simulink model "simulinkBUCK"  (R2022b)
settings: Solver=ode45  StartTime=0.0  StopTime=0.01  RelTol=1e-3
values from neighbouring files (symbols this model uses):
  C = 10e-6    (= 1e-05)    [BUCK_Parameters.m]
  L = 0.002    [BUCK_Parameters.m]
  R = 10    [BUCK_Parameters.m]
  Vin = 32    [BUCK_Parameters.m]
settings Model: Creator=ferch  LastModifiedBy=ferch

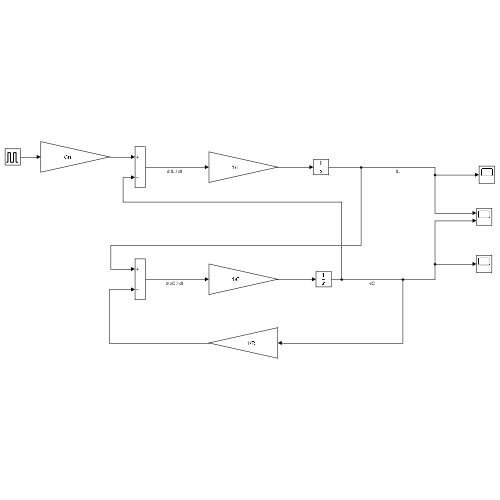
[thumbnail: Simulink's stored preview of the top-level diagram]
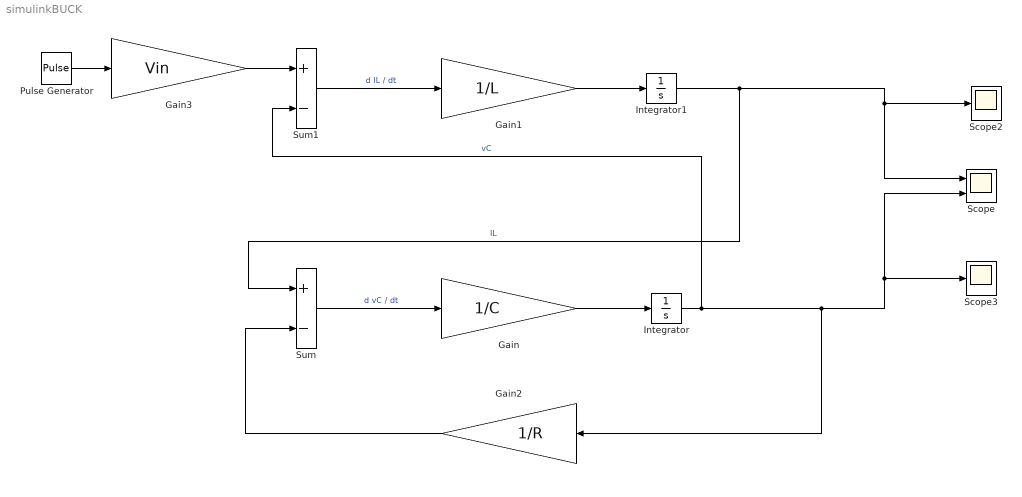
== system simulinkBUCK ==
  Gain : Gain  Gain=1/C
  Gain1 : Gain  Gain=1/L
  Gain2 : Gain  Gain=1/R
  Gain3 : Gain  Gain=Vin
  Integrator : Integrator
  Integrator1 : Integrator
  Pulse Generator : DiscretePulseGenerator  PulseType=Time based  Period=1/100e3  PulseWidth=40
  Scope : Scope  NumInputPorts=2
  Scope2 : Scope
  Scope3 : Scope
  Sum : Sum  Inputs=+-
  Sum1 : Sum  Inputs=+-
  wires:
  Gain/1 -> Integrator/1
  Sum/1 -> Gain/1  "d vC / dt"
  Sum1/1 -> Gain1/1  "d IL / dt"
  Gain1/1 -> Integrator1/1
  Integrator1/1 -> Sum/1, Scope/1, Scope2/1  "IL"
  Integrator/1 -> Gain2/1, Scope/2, Scope3/1, Sum1/2  "vC"
  Pulse Generator/1 -> Gain3/1
  Gain2/1 -> Sum/2
  Gain3/1 -> Sum1/1
